simulink model "app01_1_sound_meter"  (R2016a)
settings: Solver=FixedStepAuto  StartTime=0.0  StopTime=100  RelTol=1e-3
undefined symbols (not defined in the file): DiscIntNeverNeededParam
libraries: embdlinuxlib x1, dspstat3 x1
settings Model: SimulationMode=external  Creator=ohori  LastModifiedBy=ohori
settings SolverCC: PositivePriorityOrder=on
settings OptimizationCC: OptimizeModelRefInitCode=on  LifeSpan=1  MaxStackSize=64
settings HardwareCC: ProdBitPerPointer=32  ProdLargestAtomicInteger=Long  ProdLargestAtomicFloat=Double  ProdWordSize=32  ProdHWDeviceType=ARM Compatible->ARM Cortex  UseEmbeddedCoderFeatures=off  UseSimulinkCoderFeatures=off
settings RTWCC: SystemTargetFile=ert.tlc  HardwareBoard=Raspberry Pi  TemplateMakefile=ert_default_tmf  RTWVerbose=off  Toolchain=GNU GCC Raspberry Pi  IncludeHyperlinkInReport=on
settings CodeAppCC: ForceParamTrailComments=on  OperatorAnnotations=on  SimulinkDataObjDesc=on  SFDataObjDesc=on  MATLABFcnDesc=on  MangleLength=10  InsertBlockDesc=on  MATLABSourceComments=on
settings ERTTargetCC: SupportNonInlinedSFcns=on  SupportVariableSizeSignals=on  ExtMode=on  ExtModeMexArgs='169.254.0.2' 0 17725  ERTSrcFileBannerTemplate=codertarget_code_template.cgt  ERTHdrFileBannerTemplate=codertarget_code_template.cgt  ERTDataSrcFileTemplate=codertarget_code_template.cgt  ERTDataHdrFileTemplate=codertarget_code_template.cgt

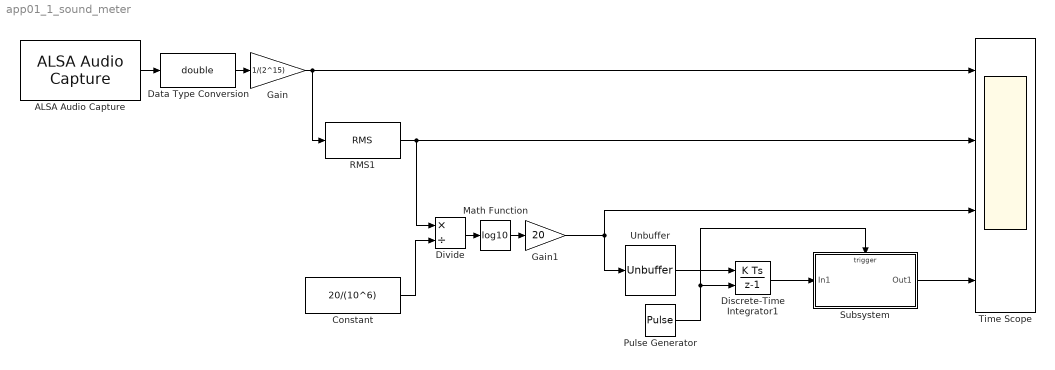
== system app01_1_sound_meter ==
  ALSA Audio Capture : embdlinuxlib/ALSA Audio Capture  deviceStr='plughw:1,0'  sampleRateEnum=44100  queueDuration=0.5  frameSize=4410  blockPlatform=Raspberry Pi
  Constant : Constant  Value=20/(10^6)
  Data Type Conversion : DataTypeConversion  OutDataTypeStr=double
  Discrete-Time Integrator1 : DiscreteIntegrator  ExternalReset=falling  InitialConditionSetting=State (most efficient)  SampleTime=-1  ICPrevOutput=DiscIntNeverNeededParam  ICPrevScaledInput=DiscIntNeverNeededParam
  Divide : Product  Inputs=*/
  Gain : Gain  Gain=1/(2^15)
  Gain1 : Gain  Gain=20
  Math Function : Math  Operator=log10  SaturateOnIntegerOverflow=on
  Pulse Generator : DiscretePulseGenerator  Period=600  SampleTime=0.1
  RMS1 : dspstat3/RMS  run=off  reset_popup=None  InputProcessing=Columns as channels (frame based)  directionMode=Each column  dimension=1
  Subsystem : Subsystem
  Time Scope : Scope  NumInputPorts=4
  Unbuffer : Unbuffer  SampleBasedProcessing=Same as frame based
  wires:
  ALSA Audio Capture/1 -> Data Type Conversion/1
  Data Type Conversion/1 -> Gain/1
  Gain/1 -> Time Scope/1, RMS1/1
  RMS1/1 -> Time Scope/2, Divide/1
  Discrete-Time Integrator1/1 -> Subsystem/1(In1)
  Pulse Generator/1 -> Subsystem/Trigger, Discrete-Time Integrator1/2
  Unbuffer/1 -> Discrete-Time Integrator1/1
  Subsystem/1(Out1) -> Time Scope/4
  Constant/1 -> Divide/2
  Divide/1 -> Math Function/1
  Math Function/1 -> Gain1/1
  Gain1/1 -> Time Scope/3, Unbuffer/1

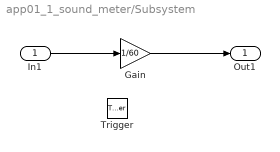
== system app01_1_sound_meter/Subsystem ==
  In1 : Inport
  Trigger : TriggerPort  VariantControl=Variant  PortDimensions=1
  Gain : Gain  Gain=1/60
  Out1 : Outport
  wires:
  In1/1 -> Gain/1
  Gain/1 -> Out1/1
